simulink model "binary_to_gray_and_back"  (R2023a)
settings: Solver=VariableStepAuto  StartTime=0.0  StopTime=0.03  RelTol=1e-3
values from neighbouring files (symbols this model uses):
  t_clock = 1/f_clock    (= 1e-08)    [uz_ssi_interface_init.m]
libraries: hdlsllib x17, simulink x1
settings Model: Creator=micha  LastModifiedBy=micha

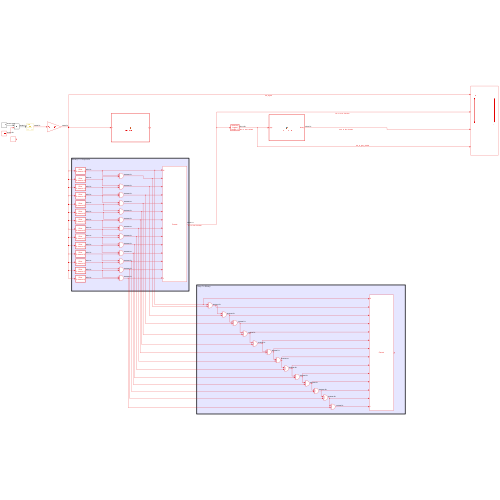
[thumbnail: Simulink's stored preview of the top-level diagram]
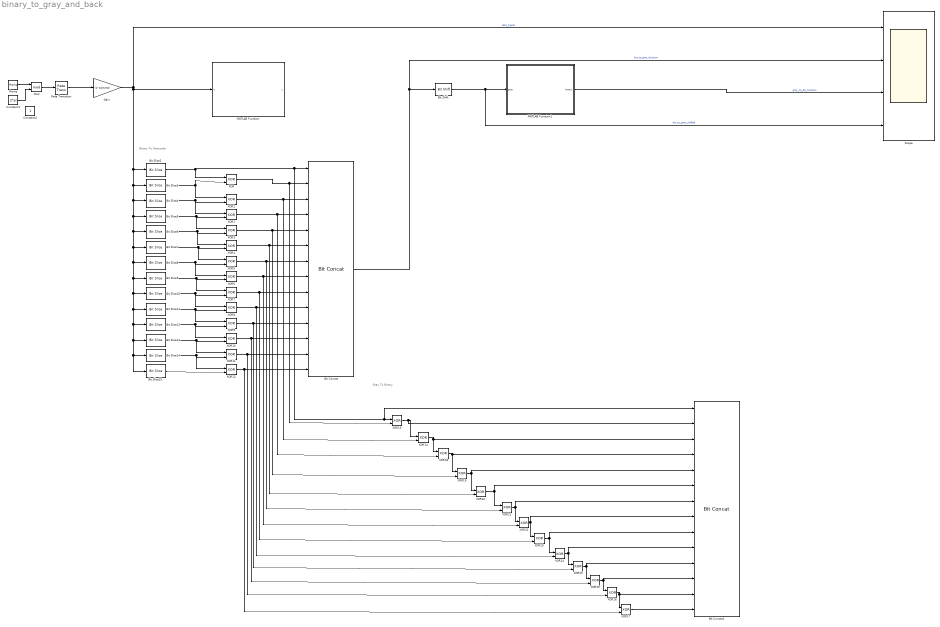
== system binary_to_gray_and_back ==
  note: Gray To Binary
  note: Binary To Graycode
  Bit Concat : hdlsllib/Logic and Bit Operations/Bit Concat  numInputs=14
  Bit Concat1 : hdlsllib/Logic and Bit Operations/Bit Concat  numInputs=14
  Bit Shift : hdlsllib/Logic and Bit Operations/Bit Shift  mode=Shift Left Logical  N=0
  Bit Slice10 : hdlsllib/Logic and Bit Operations/Bit Slice  lidx=5  ridx=5
  Bit Slice11 : hdlsllib/Logic and Bit Operations/Bit Slice  lidx=4  ridx=4
  Bit Slice12 : hdlsllib/Logic and Bit Operations/Bit Slice  lidx=3  ridx=3
  Bit Slice13 : hdlsllib/Logic and Bit Operations/Bit Slice  lidx=2  ridx=2
  Bit Slice14 : hdlsllib/Logic and Bit Operations/Bit Slice  lidx=1  ridx=1
  Bit Slice15 : hdlsllib/Logic and Bit Operations/Bit Slice  lidx=0  ridx=0
  Bit Slice2 : hdlsllib/Logic and Bit Operations/Bit Slice  lidx=13  ridx=13
  Bit Slice3 : hdlsllib/Logic and Bit Operations/Bit Slice  lidx=12  ridx=12
  Bit Slice4 : hdlsllib/Logic and Bit Operations/Bit Slice  lidx=11  ridx=11
  Bit Slice5 : hdlsllib/Logic and Bit Operations/Bit Slice  lidx=10  ridx=10
  Bit Slice6 : hdlsllib/Logic and Bit Operations/Bit Slice  lidx=9  ridx=9
  Bit Slice7 : hdlsllib/Logic and Bit Operations/Bit Slice  lidx=8  ridx=8
  Bit Slice8 : hdlsllib/Logic and Bit Operations/Bit Slice  lidx=7  ridx=7
  Bit Slice9 : hdlsllib/Logic and Bit Operations/Bit Slice  lidx=6  ridx=6
  Constant1 : Constant  Value=2*pi  SampleTime=t_clock
  Constant2 : Constant  SampleTime=t_clock
  Gain : Gain  Gain=(2^13)/(2*pi)  OutDataTypeStr=uint32
  MATLAB Function : MATLAB Function  TreatAsAtomicUnit=on
  MATLAB Function1 : MATLAB Function  TreatAsAtomicUnit=on
  Mod : Math  Operator=mod
  Ramp : simulink/Sources/Ramp  slope=-2*pi*50  start=0  InitialOutput=0
  Rate Transition : RateTransition  OutPortSampleTime=t_clock
  Scope : Scope  NumInputPorts=4
  XOR{,1..25} (26 alike) : Logic  Operator=XOR  IconShape=distinctive  AllPortsSameDT=off  OutDataTypeStr=boolean
  wires:
  Mod/1 -> Rate Transition/1
  Bit Concat/1 -> Scope/2, Bit Shift/1  "bin_to_gray_function"
  Ramp/1 -> Mod/1
  Constant1/1 -> Mod/2
  Rate Transition/1 -> Gain/1
  Gain/1 -> Bit Slice7/1, Bit Slice8/1, Bit Slice9/1, Bit Slice11/1, Bit Slice12/1, Bit Slice13/1, Bit Slice14/1, Bit Slice15/1, Bit Slice10/1, Bit Slice6/1, Bit Slice5/1, Bit Slice4/1, Bit Slice3/1, Bit Slice2/1, MATLAB Function/1(u), Scope/1  "test_signal"
  Bit Slice2/1 -> Bit Concat1/1, XOR13/1, Bit Concat/1, XOR/1
  Bit Slice3/1 -> XOR1/1, XOR/2
  XOR/1 -> XOR13/2, Bit Concat/2
  Bit Slice5/1 -> XOR3/1, XOR2/2
  Bit Slice4/1 -> XOR2/1, XOR1/2
  Bit Slice6/1 -> XOR4/1, XOR3/2
  Bit Slice10/1 -> XOR8/1, XOR7/2
  Bit Slice9/1 -> XOR7/1, XOR6/2
  Bit Slice7/1 -> XOR4/2, XOR5/1
  Bit Slice8/1 -> XOR5/2, XOR6/1
  Bit Slice11/1 -> XOR9/1, XOR8/2
  Bit Slice14/1 -> XOR11/2, XOR12/1
  Bit Slice15/1 -> XOR12/2
  Bit Slice12/1 -> XOR10/1, XOR9/2
  Bit Slice13/1 -> XOR11/1, XOR10/2
  XOR12/1 -> XOR17/2, Bit Concat/14
  XOR11/1 -> XOR16/2, Bit Concat/13
  XOR10/1 -> XOR15/2, Bit Concat/12
  XOR9/1 -> XOR25/2, Bit Concat/11
  XOR8/1 -> XOR24/2, Bit Concat/10
  XOR7/1 -> XOR23/2, Bit Concat/9
  XOR6/1 -> XOR22/2, Bit Concat/8
  XOR4/1 -> XOR20/2, Bit Concat/6
  XOR3/1 -> XOR19/2, Bit Concat/5
  XOR2/1 -> XOR18/2, Bit Concat/4
  XOR1/1 -> XOR14/2, Bit Concat/3
  XOR13/1 -> Bit Concat1/2, XOR14/1
  XOR14/1 -> Bit Concat1/3, XOR18/1
  XOR18/1 -> Bit Concat1/4, XOR19/1
  XOR19/1 -> XOR20/1, Bit Concat1/5
  XOR20/1 -> XOR21/1, Bit Concat1/6
  XOR21/1 -> XOR22/1, Bit Concat1/7
  XOR22/1 -> XOR23/1, Bit Concat1/8
  XOR23/1 -> XOR24/1, Bit Concat1/9
  XOR24/1 -> XOR25/1, Bit Concat1/10
  XOR25/1 -> XOR15/1, Bit Concat1/11
  XOR15/1 -> XOR16/1, Bit Concat1/12
  XOR16/1 -> XOR17/1, Bit Concat1/13
  XOR5/1 -> Bit Concat/7, XOR21/2
  XOR17/1 -> Bit Concat1/14
  MATLAB Function1/1(binary) -> Scope/3  "gray_to_bin_function"
  Bit Shift/1 -> Scope/4, MATLAB Function1/1(gray)  "bin_to_gray_shifted"

== matlab function binary_to_gray_and_back/MATLAB Function ==
  data: u input; y output
function y = BinaryToGray(u)
%#codegen

y = bitxor(u,(bitshift(u,-1)));

== matlab function binary_to_gray_and_back/MATLAB Function1 ==
  data: gray input; binary output
function binary = GrayToBinary(gray)
%#codegen

binary = gray;
    for i = 1:24 % 24 shifts for 25-bit word
        shift_val = bitshift(gray, -i);
        binary = bitxor(binary, shift_val);
    end

end
